simulink model "tqdtqr_rebuild_V3"  (R2021b)
settings: Solver=VariableStepAuto  StartTime=0.0  StopTime=10.0  RelTol=1e-3
undefined symbols (not defined in the file): ATQD_AfterTqMinGain_X_Deg, ATQD_APSCreepBaseTqD_X_kph, ATQD_APSCreepBaseTqD_Y_Deg, ATQD_APSCreepBaseTqR_X_kph, ATQD_APSCreepBaseTqR_Y_Deg, ATQD_APSCreepIterm_X_kph, ATQD_APSCreepIterm_Y_kph, ATQD_APSCreepPterm_X_kph, ATQD_APSCreepPterm_Y_kph, ATQD_APSDecReq_X_kph, ATQD_APSDecReq_Y_mps2, ATQD_APSDecReqCMD_X_kph, ATQD_APSDecReqTs_X_pct, ATQD_APSDecTimeGain_X_Deg, ATQD_APSDecTimeGain_Y_s, ATQD_APSReqLowSpd_X_Deg, ATQD_AutoHoldReleaseBPS_X_Deg, ATQD_AWDLoadTrqnsGain_X_kg, ATQD_AWDLoadTrqnsGain_Y_pct, ATQD_BOSEnBPSPosn_X_kph, ATQD_BOSMap_X_rpm, ATQD_BOSMap_Y_pct, ATQD_CreepBaseTqD_X_kph, ATQD_CreepBaseTqD_Y_Deg, ATQD_CreepBaseTqR_X_kph, ATQD_CreepBaseTqR_Y_Deg, ATQD_CreepBPSDisPosn_X_Deg, ATQD_CreepBPSDisPosnR_X_Deg, ATQD_CreepBPSEnPosn_X_Deg, ATQD_CreepBPSEnPosnR_X_Deg, ATQD_CreepDeltaTq_X_kph, ATQD_CreepIterm_X_kph, ATQD_CreepIterm_Y_kph, ATQD_CreepItermMaxLimit_X_pct, ATQD_CreepPreloadTime_X_kph, ATQD_CreepPreloadTq_X_kph, ATQD_CreepPreloadTq_Y_s, ATQD_CreepProtTq_X_Deg, ATQD_CreepPterm_X_kph, ATQD_CreepPterm_Y_kph, ATQD_CreepRrTqSpRat_X_rpm, ATQD_CreepRrTqSpRat_Y_Nm, ATQD_CreepTargetSpdD_X_pct, ATQD_CreepTargetSpdR_X_pct, ATQD_CreepUpLimitTq_X_rpm, ATQD_DecIneOPDHoldEnDelay_X_Deg, ATQD_DecIneOPDHoldEnDelay_Y_bar, ATQD_ECOTqMapD_X_rpm, ATQD_ECOTqMapD_Y_pct, ATQD_EMTqMapD_X_rpm, ATQD_EMTqMapD_Y_pct, ATQD_EOPDTqMapDCon_X_rpm, ATQD_EOPDTqMapDCon_Y_Deg, ATQD_EstInitVehWeight_X_c, ATQD_FAfterTqCMDGain_X_rpm, ATQD_FAfterTqCMDGain_Y_pct, ATQD_ForceLowSpd_X_Deg, ATQD_ForcePLimitSpd_X_Deg, ATQD_FrLossMAPLowV_X_rpm, ATQD_FrLossMAPLowV_Y_Nm ... (+949)
libraries: simulink x235, hcu_lib x208, tqr x63, tqd x6
(part 25 of 37)

== system tqdtqr_rebuild_V3/Input_Convert/Signal function/combo key/Mode Coordination ==
  VSCP_StreetFightMode_flg : Inport
  VSCP_EngineeringMode_flg : Inport  Port=2
  VSCP_ManufactureMode_flg : Inport  Port=3
  VSCP_ExhibitionMode_flg : Inport  Port=4
  VSCP_DiagnosisOffMode_flg : Inport  Port=5
  DiagnosisOff : Subsystem  TreatAsAtomicUnit=on
  Engineering : Subsystem  TreatAsAtomicUnit=on
  Exhibition : Subsystem  TreatAsAtomicUnit=on
  If : If  NumInputs=5  IfExpression=u1 ~=0  ElseIfExpressions=u2 ~= 0, u3 ~= 0, u4 ~= 0, u5 ~= 0
  Manufacture : Subsystem  TreatAsAtomicUnit=on
  Merge : Merge  Inputs=6
  Product : Subsystem  TreatAsAtomicUnit=on
  StreetFight : Subsystem  TreatAsAtomicUnit=on
  VSCP_SysMode_enum : Outport
  wires:
  [VSCP_ManufactureMode_flg] -> If/3
  [VSCP_StreetFightMode_flg] -> If/1
  [VSCP_DiagnosisOffMode_flg] -> If/5
  [VSCP_ExhibitionMode_flg] -> If/4
  [VSCP_EngineeringMode_flg] -> If/2
  VSCP_StreetFightMode_flg/1 -> [VSCP_StreetFightMode_flg]
  VSCP_EngineeringMode_flg/1 -> [VSCP_EngineeringMode_flg]
  VSCP_ManufactureMode_flg/1 -> [VSCP_ManufactureMode_flg]
  VSCP_ExhibitionMode_flg/1 -> [VSCP_ExhibitionMode_flg]
  VSCP_DiagnosisOffMode_flg/1 -> [VSCP_DiagnosisOffMode_flg]
  If/1 -> StreetFight/Action
  If/2 -> Engineering/Action
  If/6 -> Product/Action
  If/3 -> Manufacture/Action
  If/4 -> Exhibition/Action
  If/5 -> DiagnosisOff/Action
  StreetFight/1(StreetFight) -> Merge/1
  Engineering/1(Engineering) -> Merge/2
  Manufacture/1(Manufacture) -> Merge/3
  Exhibition/1(Exhibition) -> Merge/4
  DiagnosisOff/1(DiagnosisOff) -> Merge/5
  Product/1(Product) -> Merge/6
  Merge/1 -> [VSCP_SysMode_enum]  "VTQD_SysMode_enum"
  [VSCP_SysMode_enum] -> VSCP_SysMode_enum/1

== system tqdtqr_rebuild_V3/Input_Convert/Signal function/combo key/Operation Condition ==
  VINP_PwrSta_enum : Inport
  VINP_ShiftGearPosn_enum : Inport  Port=2
  VSCP_ComboKeyEnCMD_flg : Inport  Port=3
  AND : Logic  AllPortsSameDT=off  OutDataTypeStr=boolean
  AND1 : Logic  AllPortsSameDT=off  OutDataTypeStr=boolean
  Constant1 : Constant  Value=ENUM_POWERSTA_ON
  Constant2 : Constant  Value=ENUM_POWERSTA_READY
  Constant3 : Constant  Value=ENUM_GEARPOSNTOCAN_N
  Constant4 : Constant  Value=ENUM_GEARPOSNTOCAN_P
  Equal{,1..3} (4 alike) : RelationalOperator  Operator===  OutDataTypeStr=boolean  RndMeth=Simplest
  OR : Logic  Operator=OR  AllPortsSameDT=off  OutDataTypeStr=boolean
  OR1 : Logic  Operator=OR  AllPortsSameDT=off  OutDataTypeStr=boolean
  VSCP_ComboKeyPreEn_flg : Outport
  VSCP_ComboKeyEn_flg : Outport  Port=2
  wires:
  OR/1 -> AND/1
  Equal2/1 -> OR1/1
  Constant3/1 -> Equal3/2
  Equal/1 -> OR/1
  [VINP_ShiftGearPosn_enum] -> Equal2/1
  Constant1/1 -> Equal1/2
  Equal3/1 -> OR1/2
  Constant4/1 -> Equal2/2
  [VINP_ShiftGearPosn_enum] -> Equal3/1
  [VINP_PwrSta_enum] -> Equal/1
  Constant2/1 -> Equal/2
  [VINP_PwrSta_enum] -> Equal1/1
  Equal1/1 -> OR/2
  OR1/1 -> AND/2
  VINP_PwrSta_enum/1 -> [VINP_PwrSta_enum]
  VINP_ShiftGearPosn_enum/1 -> [VINP_ShiftGearPosn_enum]
  [VSCP_ComboKeyPreEn_flg] -> VSCP_ComboKeyPreEn_flg/1
  AND/1 -> [VSCP_ComboKeyPreEn_flg]  "VTQD_ComboKeyPreEn_flg"
  VSCP_ComboKeyEnCMD_flg/1 -> [VSCP_ComboKeyEnCMD_flg]
  [VSCP_ComboKeyPreEn_flg] -> AND1/1
  [VSCP_ComboKeyEnCMD_flg] -> AND1/2
  AND1/1 -> [VSCP_ComboKeyEn_flg]  "VTQD_ComboKeyEn_flg"
  [VSCP_ComboKeyEn_flg] -> VSCP_ComboKeyEn_flg/1

== system tqdtqr_rebuild_V3/Input_Convert/Signal function/combo key/Signal Status Detection ==
  note: Button result -> combo key command
  note: Button status
  note: Button result -> combo key value
  note: Button status
  note: Combo Key Note:
      | ENUM_COMBOKEY_NONE = uint8(0); None
      | ENUM_COMBOKEY_REGENDOWN = uint8(1); VINP_SWC2RegenDown_flg
      | ENUM_COMBOKEY_REGENUP = uint8(2); VINP_SWC2RegenUp_flg
      | ENUM_COMBOKEY_RESUP = uint8(3); VINP_SWC2LScrollUpSta_flg
      | ENUM_COMBOKEY_SETDOWN = uint8(4); VINP_SWC2LScrollDownSta_flg
      | ENUM_COMBOKEY_SWCUP = uint8(5); VINP_SWC2RScrollUpSta_flg
      | ENUM_COMBOKEY_SWCDOWN = uint8(6); VINP_SWC2RScrollDownSta_flg
      | ENUM_COMBOKEY_CANCEL = uint8(7); VINP_SWC2LScrollPressSta_flg
      | ENUM_COMBOKEY_SWCACC = uint8(8); VINP_SWC2LADASSta_flg
      | ENUM_COMBOKEY_DISTANCE = uint8(9); VINP_SWC2LDriveModeSta_flg
      | ENUM_COMBOKEY_SWCMODE = uint8(10); VINP_SWC2RScrollPressSta_flg
      | ENUM_COMBOKEY_SWCRIGHT = uint8(11); VINP_SWC2RRightSta_flg
      | ENUM_COMBOKEY_SWCLEFT = uint8(12); VINP_SWC2RLeftSta_flg
  TASK_TIME_10_MS : Inport
  VINP_SWCRegenDown_flg : Inport  Port=2
  VINP_SWCRegenUp_flg : Inport  Port=3
  VINP_SWCResUpSta_flg : Inport  Port=4
  VINP_SWCSetdownSta_flg : Inport  Port=5
  VINP_SWCUpSta_flg : Inport  Port=6
  VINP_SWCDownSta_flg : Inport  Port=7
  VINP_SWCCANCELSta_flg : Inport  Port=8
  VSCP_ComboKeyPreEn_flg : Inport  Port=9
  VINP_SWCACCSta_flg : Inport  Port=10
  VSCP_SysMode_enum : Inport  Port=11
  VINP_SWCDistanceSta_flg : Inport  Port=12
  VINP_SWCmodeSta_flg : Inport  Port=13
  VINP_SWCRightSta_flg : Inport  Port=14
  VINP_SWCLeftSta_flg : Inport  Port=15
  VSCP_ComboKeyEn_flg : Inport  Port=16
  AND{,1..14} (15 alike) : Logic  AllPortsSameDT=off  OutDataTypeStr=boolean
  Constant{,1..5,10..15} (12 alike) : Constant  Value=KTQD_SetSpdShortPLim_s
  Constant{6..9} (4 alike) : Constant  Value=KTQD_ComboKeyLongDet_s
  Delay : Delay  DelayLength=1
  DelayEnable{,1..15} (16 alike) : hcu_lib/Basic_Blocks/DelayEnable
  Detect Decrease{,1..5,10..15} (12 alike) : simulink/Logic and Bit Operations/Detect Decrease  vinit=boolean(0)  OutDataTypeStr=boolean
  Detect Decrease{6..9} (4 alike) : simulink/Logic and Bit Operations/Detect Decrease  vinit=0.0  OutDataTypeStr=boolean
  If : If  NumInputs=12  IfExpression=u1~=0  ElseIfExpressions=u2~=0,u3~=0,u4~=0,u5~=0,u6~=0,u7 ~=0,u8~=0,u9~=0,u10~=0,u11~=0,u12~=0
  Merge : Merge  Inputs=13
  None : Subsystem  TreatAsAtomicUnit=on
  SR_Latch : hcu_lib/Basic_Blocks/SR_Latch
  SWCACCSta : Subsystem  TreatAsAtomicUnit=on
  SWCCANCELStaShort : Subsystem  TreatAsAtomicUnit=on
  SWCDistanceSta : Subsystem  TreatAsAtomicUnit=on
  SWCDownStaShort : Subsystem  TreatAsAtomicUnit=on
  SWCLeftSta : Subsystem  TreatAsAtomicUnit=on
  SWCRegenDownShort : Subsystem  TreatAsAtomicUnit=on
  SWCRegenUpShort : Subsystem  TreatAsAtomicUnit=on
  SWCResUpStaShort : Subsystem  TreatAsAtomicUnit=on
  SWCRightSta : Subsystem  TreatAsAtomicUnit=on
  SWCSetdownStaShort : Subsystem  TreatAsAtomicUnit=on
  SWCUpStaShort : Subsystem  TreatAsAtomicUnit=on
  SWCmodeSta : Subsystem  TreatAsAtomicUnit=on
  Street Fight Switch Off : Subsystem
  VSCP_ComboKey_enum : Outport
  VSCP_ComboKeyEnCMD_flg : Outport  Port=2
  VSCP_ComboKeyReset_flg : Outport  Port=3
  VSCP_ComboKeyEnter_flg : Outport  Port=4
  VSCP_StreetFightModeOff_flg : Outport  Port=5
  wires:
  [VSCP_ComboKey_enum] -> VSCP_ComboKey_enum/1
  Constant/1 -> DelayEnable/2
  SWCRegenUpShort/1(SWCRegenUpShort_enum) -> [SWCRegenUpShort_enum]
  [SWCUpStaShort_enum] -> Merge/5
  VINP_SWCResUpSta_flg/1 -> [VINP_SWCResUpSta_flg]
  [VINP_SWCSetdownSta_flg] -> DelayEnable3/1
  SWCUpStaShort/1(SWCUpStaShort_enum) -> [SWCUpStaShort_enum]
  Detect Decrease3/1 -> [VSCP_SWCSetdownStaShort_flg]  "VTQD_SWCSetdownStaShort_flg"
  Detect Decrease5/1 -> [VSCP_SWCDownStaShort_flg]  "VTQD_SWCDownStaShort_flg"
  If/2 -> SWCRegenUpShort/Action
  Constant2/1 -> DelayEnable2/2
  DelayEnable4/1 -> Detect Decrease4/1
  Detect Decrease4/1 -> [VSCP_SWCUpStaShort_flg]  "VTQD_SWCUpStaShort_flg"
  DelayEnable5/1 -> Detect Decrease5/1
  Constant5/1 -> DelayEnable5/2
  If/6 -> SWCDownStaShort/Action
  [TASK_TIME_10_MS] -> DelayEnable3/3
  [SWCSetdownStaShort_enum] -> Merge/4
  [TASK_TIME_10_MS] -> DelayEnable5/3
  Constant3/1 -> DelayEnable3/2
  VINP_SWCRegenDown_flg/1 -> [VINP_SWCRegenDown_flg]
  [SWCResUpStaShort_enum] -> Merge/3
  DelayEnable3/1 -> Detect Decrease3/1
  [VINP_SWCDownSta_flg] -> DelayEnable5/1
  If/5 -> SWCUpStaShort/Action
  Detect Decrease/1 -> [VSCP_SWCRegenDownShort_flg]  "VTQD_SWCRegenDownShort_flg"
  TASK_TIME_10_MS/1 -> [TASK_TIME_10_MS]
  [TASK_TIME_10_MS] -> DelayEnable4/3
  If/13 -> None/Action
  Detect Decrease2/1 -> [VSCP_SWCResUpStaShort_flg]  "VTQD_SWCResUpStaShort_flg"
  If/4 -> SWCSetdownStaShort/Action
  Detect Decrease1/1 -> [VSCP_SWCRegenUpShort_flg]  "VTQD_SWCRegenUpShort_flg"
  VINP_SWCDownSta_flg/1 -> [VINP_SWCDownSta_flg]
  [VINP_SWCUpSta_flg] -> DelayEnable4/1
  Constant4/1 -> DelayEnable4/2
  [SWCRegenUpShort_enum] -> Merge/2
  If/1 -> SWCRegenDownShort/Action
  Constant1/1 -> DelayEnable1/2
  [TASK_TIME_10_MS] -> DelayEnable/3
  VINP_SWCSetdownSta_flg/1 -> [VINP_SWCSetdownSta_flg]
  [VINP_SWCRegenDown_flg] -> DelayEnable/1
  [SWCDownStaShort_enum] -> Merge/6
  VINP_SWCRegenUp_flg/1 -> [VINP_SWCRegenUp_flg]
  DelayEnable/1 -> Detect Decrease/1
  [VINP_SWCResUpSta_flg] -> DelayEnable2/1
  [TASK_TIME_10_MS] -> DelayEnable2/3
  DelayEnable2/1 -> Detect Decrease2/1
  VINP_SWCUpSta_flg/1 -> [VINP_SWCUpSta_flg]
  [SWCRegenDownShort_enum] -> Merge/1
  None/1(None_enum) -> [None_enum]
  [VINP_SWCRegenUp_flg] -> DelayEnable1/1
  [TASK_TIME_10_MS] -> DelayEnable1/3
  DelayEnable1/1 -> Detect Decrease1/1
  If/3 -> SWCResUpStaShort/Action
  SWCRegenDownShort/1(SWCRegenDownShort_enum) -> [SWCRegenDownShort_enum]
  SWCResUpStaShort/1(SWCResUpStaShort_enum) -> [SWCResUpStaShort_enum]
  SWCSetdownStaShort/1(SWCSetdownStaShort_enum) -> [SWCSetdownStaShort_enum]
  Merge/1 -> [VSCP_ComboKey_enum]  "VTQD_ComboKey_enum"
  SWCDownStaShort/1(SWCDownStaShort_enum) -> [SWCDownStaShort_enum]
  [VINP_SWCRegenDown_flg] -> DelayEnable6/1
  [TASK_TIME_10_MS] -> DelayEnable6/3
  Constant6/1 -> DelayEnable6/2
  DelayEnable6/1 -> [VSCP_SWCRegenDownLong_flg]  "VTQD_SWCRegenDownLong_flg"
  DelayEnable7/1 -> [VSCP_SWCRegenUpLong_flg]  "VTQD_SWCRegenUpLong_flg"
  Constant7/1 -> DelayEnable7/2
  [TASK_TIME_10_MS] -> DelayEnable7/3
  [VINP_SWCRegenUp_flg] -> DelayEnable7/1
  [VSCP_SWCRegenDownLong_flg] -> AND/1
  [VSCP_SWCRegenUpLong_flg] -> AND/2
  SR_Latch/1 -> [VSCP_ComboKeyEnCMD_flg]  "VTQD_ComboKeyEnCMD_flg"
  VINP_SWCCANCELSta_flg/1 -> [VINP_SWCCANCELSta_flg]
  [VINP_SWCCANCELSta_flg] -> DelayEnable8/1
  [TASK_TIME_10_MS] -> DelayEnable8/3
  Constant8/1 -> DelayEnable8/2
  DelayEnable8/1 -> [VSCP_SWCCANCELStaLong_flg]  "VTQD_SWCCANCELStaLong_flg"
  [VSCP_ComboKeyEnCMD_flg] -> VSCP_ComboKeyEnCMD_flg/1
  AND/1 -> Detect Decrease6/1
  Detect Decrease6/1 -> SR_Latch/1
  [VSCP_SWCCANCELStaLong_flg] -> Detect Decrease7/1
  Detect Decrease7/1 -> SR_Latch/2
  VSCP_ComboKeyPreEn_flg/1 -> [VSCP_ComboKeyPreEn_flg]
  AND1/1 -> If/1
  [VSCP_ComboKeyPreEn_flg] -> AND1/2
  AND2/1 -> If/2
  [VSCP_ComboKeyPreEn_flg] -> AND2/2
  AND3/1 -> If/3
  [VSCP_SWCResUpStaShort_flg] -> AND3/1
  [VSCP_ComboKeyPreEn_flg] -> AND3/2
  AND4/1 -> If/4
  [VSCP_ComboKeyPreEn_flg] -> AND4/2
  AND5/1 -> If/5
  [VSCP_ComboKeyPreEn_flg] -> AND5/2
  AND6/1 -> If/6
  [VSCP_ComboKeyPreEn_flg] -> AND6/2
  DelayEnable9/1 -> [VSCP_SWCACCStaLong_flg]  "VTQD_SWCACCStaLong_flg"
  Constant9/1 -> DelayEnable9/2
  [TASK_TIME_10_MS] -> DelayEnable9/3
  [VINP_SWCACCSta_flg] -> DelayEnable9/1
  VINP_SWCACCSta_flg/1 -> [VINP_SWCACCSta_flg]
  [VSCP_SWCACCStaLong_flg] -> Detect Decrease8/1
  [VSCP_ComboKeyReset_flg] -> VSCP_ComboKeyReset_flg/1
  [VSCP_SWCCANCELStaLong_flg] -> Detect Decrease9/1
  [VSCP_ComboKeyEnter_flg] -> VSCP_ComboKeyEnter_flg/1
  Detect Decrease8/1 -> AND7/1
  [VSCP_ComboKeyEn_flg] -> AND7/2
  AND7/1 -> [VSCP_ComboKeyReset_flg]  "VTQD_ComboKeyReset_flg"
  Detect Decrease9/1 -> AND8/1
  AND8/1 -> [VSCP_ComboKeyEnter_flg]  "VTQD_ComboKeyEnter_flg"
  [VINP_SWCCANCELSta_flg] -> DelayEnable10/1
  [TASK_TIME_10_MS] -> DelayEnable10/3
  Constant10/1 -> DelayEnable10/2
  DelayEnable10/1 -> Detect Decrease10/1
  Detect Decrease10/1 -> [VSCP_SWCCANCELStaShort_flg]  "VTQD_SWCCANCELStaShort_flg"
  Street Fight Switch Off/1(VSCP_StreetFightModeOff_flg) -> [VSCP_StreetFightModeOff_flg]
  [TASK_TIME_10_MS] -> Street Fight Switch Off/1(TASK_TIME_10_MS)
  [VSCP_SWCCANCELStaShort_flg] -> Street Fight Switch Off/2(VSCP_SWCCANCELStaShort_flg)
  [VSCP_ComboKeyPreEn_flg] -> Street Fight Switch Off/3(VSCP_ComboKeyPreEn_flg)
  [VSCP_SWCCANCELStaLong_flg] -> Street Fight Switch Off/4(SWCCANCELStaLong_flg)
  [VSCP_StreetFightModeOff_flg] -> VSCP_StreetFightModeOff_flg/1
  VSCP_SysMode_enum/1 -> [VSCP_SysMode_enum]
  [VSCP_SysMode_enum] -> Street Fight Switch Off/5(VSCP_SysMode_enum)
  Detect Decrease11/1 -> [VSCP_SWCACCSta_flg]  "VSCP_SWCACCSta_flg"
  DelayEnable11/1 -> Detect Decrease11/1
  Constant11/1 -> DelayEnable11/2
  [TASK_TIME_10_MS] -> DelayEnable11/3
  [VINP_SWCACCSta_flg] -> DelayEnable11/1
  [VSCP_ComboKeyPreEn_flg] -> AND9/2
  AND9/1 -> If/7
  SWCCANCELStaShort/1(SWCCANCELStaShort_enum) -> [SWCCANCELStaShort_enum]
  If/7 -> SWCCANCELStaShort/Action
  [VSCP_ComboKeyPreEn_flg] -> AND10/2
  AND10/1 -> If/8
  SWCACCSta/1(SWCACCSta_enum) -> [SWCACCSta_enum]
  If/8 -> SWCACCSta/Action
  VINP_SWCDistanceSta_flg/1 -> [VINP_SWCDistanceSta_flg]
  [VINP_SWCDistanceSta_flg] -> DelayEnable12/1
  [TASK_TIME_10_MS] -> DelayEnable12/3
  Constant12/1 -> DelayEnable12/2
  DelayEnable12/1 -> Detect Decrease12/1
  Detect Decrease12/1 -> [VSCP_SWCDistanceSta_flg]  "VTQD_SWCDistanceSta_flg"
  [VSCP_ComboKeyPreEn_flg] -> AND11/2
  AND11/1 -> If/9
  If/9 -> SWCDistanceSta/Action
  SWCDistanceSta/1(SWCDownStaShort_enum) -> [SWCDistanceSta_enum]
  VINP_SWCmodeSta_flg/1 -> [VINP_SWCmodeSta_flg]
  Detect Decrease13/1 -> [VSCP_SWCmodeSta_flg]  "VTQD_SWCmodeSta_flg"
  DelayEnable13/1 -> Detect Decrease13/1
  Constant13/1 -> DelayEnable13/2
  [TASK_TIME_10_MS] -> DelayEnable13/3
  [VINP_SWCmodeSta_flg] -> DelayEnable13/1
  [VSCP_ComboKeyPreEn_flg] -> AND12/2
  AND12/1 -> If/10
  If/10 -> SWCmodeSta/Action
  SWCmodeSta/1(SWCmodeSta_enum) -> [SWCmodeSta_enum]
  VINP_SWCRightSta_flg/1 -> [VINP_SWCRightSta_flg]
  [VINP_SWCRightSta_flg] -> DelayEnable14/1
  [TASK_TIME_10_MS] -> DelayEnable14/3
  Constant14/1 -> DelayEnable14/2
  DelayEnable14/1 -> Detect Decrease14/1
  Detect Decrease14/1 -> [VSCP_SWCRightSta_flg]  "VTQD_SWCRightSta_flg"
  [VSCP_ComboKeyPreEn_flg] -> AND13/2
  AND13/1 -> If/11
  If/11 -> SWCRightSta/Action
  SWCRightSta/1(SWCRightSta_enum) -> [SWCRightSta_enum]
  VINP_SWCLeftSta_flg/1 -> [VINP_SWCLeftSta_flg]
  Detect Decrease15/1 -> [VSCP_SWCLeftSta_flg]  "VTQD_SWCLeftSta_flg"
  DelayEnable15/1 -> Detect Decrease15/1
  Constant15/1 -> DelayEnable15/2
  [TASK_TIME_10_MS] -> DelayEnable15/3
  [VINP_SWCLeftSta_flg] -> DelayEnable15/1
  [VSCP_ComboKeyPreEn_flg] -> AND14/2
  AND14/1 -> If/12
  If/12 -> SWCLeftSta/Action
  SWCLeftSta/1(SWCLeftSta_enum) -> [SWCLeftSta_enum]
  [None_enum] -> Merge/13
  [SWCCANCELStaShort_enum] -> Merge/7
  [SWCACCSta_enum] -> Merge/8
  [SWCDistanceSta_enum] -> Merge/9
  [SWCmodeSta_enum] -> Merge/10
  [SWCRightSta_enum] -> Merge/11
  [SWCLeftSta_enum] -> Merge/12
  [VSCP_SWCRegenDownShort_flg] -> AND1/1
  [VSCP_SWCRegenUpShort_flg] -> AND2/1
  [VSCP_SWCSetdownStaShort_flg] -> AND4/1
  [VSCP_SWCUpStaShort_flg] -> AND5/1
  [VSCP_SWCDownStaShort_flg] -> AND6/1
  [VSCP_SWCCANCELStaShort_flg] -> AND9/1
  [VSCP_SWCACCSta_flg] -> AND10/1
  [VSCP_SWCDistanceSta_flg] -> AND11/1
  [VSCP_SWCmodeSta_flg] -> AND12/1
  [VSCP_SWCRightSta_flg] -> AND13/1
  [VSCP_SWCLeftSta_flg] -> AND14/1
  VSCP_ComboKeyEn_flg/1 -> [VSCP_ComboKeyEn_flg]
  Delay/1 -> AND8/2
  [VSCP_ComboKeyEn_flg] -> Delay/1

== system tqdtqr_rebuild_V3/Input_Convert/Main function/AvaliableTqLimit function/TorqueCapacityCalcalation/CapacityDistribution ==
  VTQD_FrEDUSpRat_cmd : Inport
  VTQD_RrEDUSpRat_rat : Inport  Port=2
  VTQD_TMPwrAvailDchrg_kW : Inport  Port=3
  VINP_HVBPwrAvailChrg_kw : Inport  Port=4
  VTQD_MotorLossTotal_kw : Inport  Port=5
  Abs1 : Abs
  Add : Sum  Inputs=+-
  Constant12 : Constant  Value=ZERO_FLOAT
  Max : MinMax  Function=max  Inputs=2
  Product{,1,4..5} (4 alike) : Product
  VTQD_FrHVBPwrAvailDchrg_kw : Outport
  VTQD_RrHVBPwrAvailDchrg_kw : Outport  Port=2
  VTQD_FrHVBPwrAvailChrg_kw : Outport  Port=3
  VTQD_RrHVBPwrAvailChrg_kw : Outport  Port=4
  wires:
  VTQD_RrEDUSpRat_rat/1 -> [VTQD_RrEDUSpRat_rat]
  VTQD_FrEDUSpRat_cmd/1 -> [VTQD_FrEDUSpRat_rat]
  VINP_HVBPwrAvailChrg_kw/1 -> Abs1/1
  Product4/1 -> VTQD_FrHVBPwrAvailChrg_kw/1
  Product5/1 -> VTQD_RrHVBPwrAvailChrg_kw/1
  Product1/1 -> VTQD_RrHVBPwrAvailDchrg_kw/1  "VTQD_RrHVBPwrAvailDchrg_kW"
  [VTQD_FrEDUSpRat_rat] -> Product4/1
  [VTQD_FrEDUSpRat_rat] -> Product/1
  Abs1/1 -> Product4/2, Product5/1
  [VTQD_RrEDUSpRat_rat] -> Product5/2
  Product/1 -> VTQD_FrHVBPwrAvailDchrg_kw/1  "VTQD_FrHVBPwrAvailDchrg_kW"
  [VTQD_RrEDUSpRat_rat] -> Product1/2
  VTQD_TMPwrAvailDchrg_kW/1 -> Add/1
  VTQD_MotorLossTotal_kw/1 -> Add/2
  Add/1 -> Max/1
  Constant12/1 -> Max/2
  Max/1 -> Product1/1, Product/2

== system tqdtqr_rebuild_V3/Input_Convert/Main function/AvaliableTqLimit function/TorqueCapacityCalcalation/MOTOR Loss MAP  ==
  note: Rear Loss Power Calculation
  note: Calabration Parameters/Maps
  note: Front Loss Power Calculation
  note: Determination
  VTQD_FrShaftSpd_rpm : Inport
  VTQD_RrShaftSpd_rpm : Inport  Port=2
  VTQD_CoordWhlTqDemFr_Nm : Inport  Port=3
  VTQD_CoordWhlTqDemRr_Nm : Inport  Port=4
  VINP_FrMCUDCBusVolt_V : Inport  Port=5
  VINP_RrMCUDCBusVolt_V : Inport  Port=6
  VPMM_DrivetrainSelect_enum : Inport  Port=7
  AND : Logic  AllPortsSameDT=off  OutDataTypeStr=boolean
  AND2 : Logic  AllPortsSameDT=off  OutDataTypeStr=boolean
  Add : Sum
  Add2 : Sum
  Add3 : Sum
  Constant : Constant  Value=KTQD_FrLossMAPLowV_V
  Constant1 : Constant  Value=KTQD_FrLossMAPHighV_V
  Constant10 : Constant  Value=eps  OutDataTypeStr=single
  Constant{6,11..13} (4 alike) : Constant  Value=ZERO_FLOAT
  Constant2 : Constant  Value=KTQD_RrLossMAPLowV_V
  Constant3 : Constant  Value=KTQD_RrLossMAPHighV_V
  Constant4 : Constant  Value=ENUM_DRIVETRAIN_AWD
  Constant5 : Constant  Value=ENUM_DRIVETRAIN_RWD
  Constant7 : Constant  Value=eps  OutDataTypeStr=single
  Divide : Product  Inputs=*/
  Divide2 : Product  Inputs=*/
  Equal : RelationalOperator  Operator===  OutDataTypeStr=boolean  RndMeth=Simplest
  Equal1 : RelationalOperator  Operator===  OutDataTypeStr=boolean  RndMeth=Simplest
  GreaterThan : RelationalOperator  Operator=>  OutDataTypeStr=boolean  RndMeth=Simplest
  GreaterThan2 : RelationalOperator  Operator=>  OutDataTypeStr=boolean  RndMeth=Simplest
  Less Than : RelationalOperator  Operator=<  OutDataTypeStr=boolean  RndMeth=Simplest
  Less Than2 : RelationalOperator  Operator=<  OutDataTypeStr=boolean  RndMeth=Simplest
  MTQD_FrLossMAPHighV_Z_kW : Lookup_n-D  BreakpointsForDimension1=ATQD_FrLossMAPLowV_Y_Nm  BreakpointsForDimension2=ATQD_FrLossMAPLowV_X_rpm  Table=MTQD_FrLossMAPHighV_Z_kW  InternalRulePriority=Speed  RndMeth=Simplest  InputSameDT=on
      settings: InputPortMap=u0,u1
  MTQD_FrLossMAPLowV_Z_kW : Lookup_n-D  BreakpointsForDimension1=ATQD_FrLossMAPLowV_Y_Nm  BreakpointsForDimension2=ATQD_FrLossMAPLowV_X_rpm  Table=MTQD_FrLossMAPLowV_Z_kW  InternalRulePriority=Speed  RndMeth=Simplest  InputSameDT=on
      settings: InputPortMap=u0,u1
  MTQD_RrLossMAPHighV_Z_kW : Lookup_n-D  BreakpointsForDimension1=ATQD_RrLossMAPLowV_Y_Nm  BreakpointsForDimension2=ATQD_RrLossMAPLowV_X_rpm  Table=MTQD_RrLossMAPHighV_Z_kW  InternalRulePriority=Speed  RndMeth=Simplest  InputSameDT=on
      settings: InputPortMap=u0,u1
  MTQD_RrLossMAPLowV_Z_kW : Lookup_n-D  BreakpointsForDimension1=ATQD_RrLossMAPLowV_Y_Nm  BreakpointsForDimension2=ATQD_RrLossMAPLowV_X_rpm  Table=MTQD_RrLossMAPLowV_Z_kW  InternalRulePriority=Speed  RndMeth=Simplest  InputSameDT=on
      settings: InputPortMap=u0,u1
  Max : MinMax  Function=max  Inputs=2
  Max1 : MinMax  Function=max  Inputs=2
  Product : Product
  Product2 : Product
  Subtract{,1..2,6..8} (6 alike) : Sum  Inputs=+-
  Switch : Switch  Criteria=u2 > Threshold
  Switch1 : Switch  Criteria=u2 > Threshold
  Switch3 : Switch  Criteria=u2 ~= 0
  Switch4 : Switch  Criteria=u2 ~= 0
  VTQD_MotorLossTotal_kW : Outport
  wires:
  VINP_FrMCUDCBusVolt_V/1 -> [VINP_FrMCUDCBusVolt_V]
  VINP_RrMCUDCBusVolt_V/1 -> [VINP_RrMCUDCBusVolt_V]
  VTQD_CoordWhlTqDemFr_Nm/1 -> [VTQD_CoordWhlTqDemFr_Nm]
  VTQD_FrShaftSpd_rpm/1 -> [VTQD_FrShaftSpd_rpm]
  VTQD_RrShaftSpd_rpm/1 -> [VTQD_RrShaftSpd_rpm]
  VTQD_CoordWhlTqDemRr_Nm/1 -> [VTQD_CoordWhlTqDemRr_Nm]
  VPMM_DrivetrainSelect_enum/1 -> [VPMM_DrivetrainSelect_enum]
  MTQD_FrLossMAPLowV_Z_kW/1 -> [VTQD_FrLossMAPLowV_kW]  "VTQD_FrLossMAPLowV_kW"
  [VTQD_RrShaftSpd_rpm] -> MTQD_RrLossMAPHighV_Z_kW/2
  Switch/1 -> [VTQD_MotorLossTotal_kW]  "VTQD_MotorLossTotal_kW"
  Add/1 -> Switch3/1
  Constant2/1 -> [VTQD_RrLossMAPLowV_V]  "VTQD_RrLossMAPLowV_V"
  Constant7/1 -> Max1/2
  Subtract/1 -> Divide/1
  Constant1/1 -> [VTQD_FrLossMAPHighV_V]  "VTQD_FrLossMAPHighV_V"
  [VTQD_RrShaftSpd_rpm] -> MTQD_RrLossMAPLowV_Z_kW/2
  Subtract8/1 -> Product2/2
  Constant3/1 -> [VTQD_RrLossMAPHighV_V]  "VTQD_RrLossMAPHighV_V"
  Subtract1/1 -> Max/1
  Constant/1 -> [VTQD_FrLossMAPLowV_V]  "VTQD_FrLossMAPLowV_V"
  [VTQD_FrLossMAPLowV_V] -> Subtract/2
  [VTQD_RrLossMAPLowV_kW] -> Subtract8/2
  Add2/1 -> Switch/1
  [VINP_RrMCUDCBusVolt_V] -> Less Than2/1
  MTQD_RrLossMAPHighV_Z_kW/1 -> [VTQD_RrLossMAPHighV_kW]  "VTQD_RrLossMAPHighV_kW"
  Switch3/1 -> [VTQD_FrLossMAPFinal_kW]  "VTQD_FrLossMAPFinal_kW"
  [VTQD_CoordWhlTqDemRr_Nm] -> GreaterThan2/1
  [VTQD_RrLossMAPHighV_kW] -> Subtract8/1
  Product/1 -> Add/1
  Divide/1 -> Product/1
  [VPMM_DrivetrainSelect_enum] -> Equal/1
  [VINP_FrMCUDCBusVolt_V] -> Subtract/1
  Max1/1 -> Divide2/2
  [VTQD_FrLossMAPLowV_kW] -> Add/2
  [VTQD_RrLossMAPHighV_V] -> Less Than2/2
  Constant4/1 -> Equal/2
  Less Than/1 -> AND/2
  [VTQD_RrLossMAPLowV_kW] -> Add3/2
  [VPMM_DrivetrainSelect_enum] -> Equal1/1
  [VINP_FrMCUDCBusVolt_V] -> Less Than/1
  Equal1/1 -> Switch1/2
  [VTQD_CoordWhlTqDemFr_Nm] -> GreaterThan/1
  GreaterThan/1 -> AND/1
  Equal/1 -> Switch/2
  AND2/1 -> Switch4/2
  Subtract2/1 -> Product/2
  [VTQD_CoordWhlTqDemFr_Nm] -> MTQD_FrLossMAPLowV_Z_kW/1
  Constant11/1 -> Switch3/3
  [VTQD_FrLossMAPHighV_kW] -> Subtract2/1
  AND/1 -> Switch3/2
  [VTQD_FrLossMAPHighV_V] -> Subtract1/1
  [VTQD_CoordWhlTqDemFr_Nm] -> MTQD_FrLossMAPHighV_Z_kW/1
  Constant10/1 -> Max/2
  [VTQD_CoordWhlTqDemRr_Nm] -> MTQD_RrLossMAPLowV_Z_kW/1
  [VTQD_CoordWhlTqDemRr_Nm] -> MTQD_RrLossMAPHighV_Z_kW/1
  MTQD_RrLossMAPLowV_Z_kW/1 -> [VTQD_RrLossMAPLowV_kW]  "VTQD_RrLossMAPLowV_kW"
  [VTQD_FrShaftSpd_rpm] -> MTQD_FrLossMAPHighV_Z_kW/2
  Constant13/1 -> GreaterThan2/2
  [VTQD_FrShaftSpd_rpm] -> MTQD_FrLossMAPLowV_Z_kW/2
  [VTQD_RrLossMAPHighV_V] -> Subtract7/1
  Constant6/1 -> GreaterThan/2
  [VTQD_FrLossMAPLowV_V] -> Subtract1/2
  Max/1 -> Divide/2
  [VTQD_FrLossMAPLowV_kW] -> Subtract2/2
  [VTQD_FrLossMAPFinal_kW] -> Switch1/3
  Subtract7/1 -> Max1/1
  [VTQD_FrLossMAPHighV_V] -> Less Than/2
  [VTQD_RrLossMAPLowV_V] -> Subtract7/2
  Add3/1 -> Switch4/1
  Product2/1 -> Add3/1
  Switch1/1 -> Switch/3
  Constant12/1 -> Switch4/3
  Divide2/1 -> Product2/1
  Constant5/1 -> Equal1/2
  [VTQD_RrLossMAPLowV_V] -> Subtract6/2
  Subtract6/1 -> Divide2/1
  [VINP_RrMCUDCBusVolt_V] -> Subtract6/1
  Switch4/1 -> [VTQD_RrLossMAPFinal_kW]  "VTQD_RrLossMAPFinal_kW"
  MTQD_FrLossMAPHighV_Z_kW/1 -> [VTQD_FrLossMAPHighV_kW]  "VTQD_FrLossMAPHighV_kW"
  [VTQD_FrLossMAPFinal_kW] -> Add2/1
  [VTQD_RrLossMAPFinal_kW] -> Switch1/1
  GreaterThan2/1 -> AND2/1
  Less Than2/1 -> AND2/2
  [VTQD_RrLossMAPFinal_kW] -> Add2/2
  [VTQD_MotorLossTotal_kW] -> VTQD_MotorLossTotal_kW/1

== system tqdtqr_rebuild_V3/Input_Convert/Main function/AvaliableTqLimit function/TorqueCapacityCalcalation/TMAvailablePwr_Calculation ==
  VINP_HVBPwrAvailDchrg_kw : Inport
  Add : Sum
  Constant : Constant  Value=KTQD_DCDCCalPwrAvailRsv_kW
  Constant1 : Constant  Value=KTQD_THCMCalPwrAvailRsv_kW
  Constant2 : Constant  Value=KTQD_TMPwrAvailDchrg_kW_ovrdflg
  Constant3 : Constant  Value=ZERO_FLOAT
  Min : MinMax  Function=max  Inputs=2
  Subtract : Sum  Inputs=+-
  Switch : Switch  Criteria=u2 ~= 0
      settings: AttributesFormatString=<%<Criteria>>
  VTQD_TMPwrAvailDchrg_kW : Outport
  wires:
  Constant3/1 -> Min/2
  Min/1 -> Switch/1
  Switch/1 -> VTQD_TMPwrAvailDchrg_kW/1  "VTQD_TMPwrAvailDchrg_kW"
  Constant2/1 -> Switch/2
  Subtract/1 -> Min/1
  Add/1 -> Subtract/2
  VINP_HVBPwrAvailDchrg_kw/1 -> Subtract/1, Switch/3
  Constant1/1 -> Add/2
  Constant/1 -> Add/1

== system tqdtqr_rebuild_V3/Input_Convert/Main function/DriverWhlTqDem function/Creep/If Action Subsystem ==
  In1 : Inport
  Action Port : ActionPort  ActionPortLabel=if(u1 ~= 0)
  Out1 : Outport
  wires:
  In1/1 -> Out1/1

== system tqdtqr_rebuild_V3/Input_Convert/Main function/DriverWhlTqDem function/Creep/If Action Subsystem1 ==
  VTQD_CreepPICtrlReset_flg : Inport
  VTQD_CreepPtermInp_c : Inport  Port=2
  VTQD_CreepItermInp_c : Inport  Port=3
  VTQD_CreepDeltaTq_Nm : Inport  Port=4
  VTQD_ActBPSPosn_pct : Inport  Port=5
  VVMC_APSActive_flg : Inport  Port=6
  Add : Sum
  Add1 : Sum  Inputs=+++
  Constant : Constant  Value=ZERO_FLOAT
  Constant1 : Constant  Value=KTQD_CreepItermMinLimit_Nm
  Constant2 : Constant  Value=KTQD_APSCreepItermMaxLim_Nm
  Constant3 : Constant  Value=ONE_FLOAT
  Constant4 : Constant  Value=ZERO_FLOAT
  Constant5 : Constant  Value=ONE_FLOAT
  Constant87 : Constant  Value=KTQD_APSCreepParOvrd_flg
  Data Type Conversion : DataTypeConversion
  MTQD_CreepItermMaxLimit_Y_Nm : Lookup_n-D  NumberOfTableDimensions=1  BreakpointsForDimension1=ATQD_CreepItermMaxLimit_X_pct  Table=MTQD_CreepItermMaxLimit_Y_Nm  ExtrapMethod=Clip  InternalRulePriority=Speed  RndMeth=Simplest  InputSameDT=on
  OR19 : Logic  Operator=OR  AllPortsSameDT=off  OutDataTypeStr=boolean
  Product : Product
  Product2 : Product
  Saturation Dynamic : simulink/Discontinuities/Saturation Dynamic  OutMin=[]  OutMax=[]  OutDataTypeStr=Inherit: Same as second input  OutDataType=fixdt(1, 16)  OutScaling=2^-10  DoSatur=off
  Switch : Switch  Criteria=u2 ~= 0
      settings: AttributesFormatString=%<Criteria>
  Switch1 : Switch  Criteria=u2 ~= 0
  Switch4 : Switch  Criteria=u2 ~= 0
      settings: AttributesFormatString=%<Criteria>
  Unit Delay : UnitDelay  InitialCondition=boolean(0)  SampleTime=-1  HasFrameUpgradeWarning=on
      settings: AttributesFormatString=%<InitialCondition>
  VTQD_CreepTotalOfstTq_Nm : Outport
  wires:
  Add1/1 -> VTQD_CreepTotalOfstTq_Nm/1  "VTQD_CreepTotalOfstTq_Nm"
  VTQD_CreepDeltaTq_Nm/1 -> [VTQD_CreepDeltaTq_Nm]
  VTQD_CreepItermInp_c/1 -> [VTQD_CreepItermInp_c]
  VTQD_CreepPtermInp_c/1 -> [VTQD_CreepPtermInp_c]
  VTQD_ActBPSPosn_pct/1 -> [VTQD_ActBPSPosn_pct]
  Data Type Conversion/1 -> Add1/3  "VTQD_CreepOffsetTq_Nm"
  Constant1/1 -> Saturation Dynamic/3
  [VTQD_ActBPSPosn_pct] -> MTQD_CreepItermMaxLimit_Y_Nm/1
  [VTQD_CreepPICtrlReset_flg] -> Switch4/2
  Constant/1 -> Switch1/1
  Product/1 -> Switch1/3
  [VTQD_CreepPtermInp_c] -> Product/1
  Constant5/1 -> Product/2
  [VTQD_CreepPICtrlReset_flg] -> Switch1/2
  Add/1 -> Switch4/3
  Switch1/1 -> Add1/1  "VTQD_CreepPtermTq_Nm"
  Saturation Dynamic/1 -> Add1/2  "VTQD_CreepItermTq_Nm"
  Product2/1 -> Add/1
  Switch4/1 -> Unit Delay/1, Saturation Dynamic/2
  Unit Delay/1 -> Add/2
  Constant4/1 -> Switch4/1
  [VTQD_CreepItermInp_c] -> Product2/2
  [VTQD_CreepDeltaTq_Nm] -> Data Type Conversion/1
  VVMC_APSActive_flg/1 -> [VVMC_APSActive_flg]
  MTQD_CreepItermMaxLimit_Y_Nm/1 -> Switch/3
  Switch/1 -> Saturation Dynamic/1  "VTQD_CreepItermMaxLimit_Nm"
  Constant87/1 -> OR19/2
  [VVMC_APSActive_flg] -> OR19/1
  OR19/1 -> Switch/2
  Constant2/1 -> Switch/1
  Constant3/1 -> Product2/1
  VTQD_CreepPICtrlReset_flg/1 -> [VTQD_CreepPICtrlReset_flg]

== system tqdtqr_rebuild_V3/Input_Convert/Main function/DriverWhlTqDem function/Creep/Switch Case Action Subsystem ==
  In1 : Inport
  Action Port : ActionPort  ActionPortLabel=elseif(u2 ~= 0)
  Out1 : Outport
  wires:
  In1/1 -> Out1/1

== system tqdtqr_rebuild_V3/Input_Convert/Main function/DriverWhlTqDem function/Driver mode determination/LHM ==
  VTQD_ActAPSPosn_pct : Inport
  VTQD_TqTargetShaftSpd_rpm : Inport  Port=2
  VTQD_GearActualPosn_enum : Inport  Port=3
  VDDM_VehMalfunLevel_enum : Inport  Port=4
  VVMC_EstSlope_Deg : Inport  Port=5
  VTQD_VehActSpd_kph : Inport  Port=6
  Enable : EnablePort
  Constant : Constant  Value=ZERO_FLOAT
  Constant1 : Constant  Value=ENUM_GEARACTUALPOSN_D
  Constant2 : Constant  Value=ENUM_GEARACTUALPOSN_R
  Constant3 : Constant  Value=ENUM_VEHMALFUNLEVEL_LEVEL2
  Constant5 : Constant  Value=ZERO_FLOAT
  Constant6 : Constant  Value=ZERO_FLOAT
  Equal1 : RelationalOperator  Operator===  OutDataTypeStr=boolean  RndMeth=Simplest
  Equal2 : RelationalOperator  Operator===  OutDataTypeStr=boolean  RndMeth=Simplest
  MTQD_LHMGrade2TqUpLim_Z_Nm : Lookup_n-D  BreakpointsForDimension1=ATQD_LHMGrade2TqUpLim_Y_Deg  BreakpointsForDimension2=ATQD_LHMGrade2TqUpLim_X_kph  Table=MTQD_LHMGrade2TqUpLim_Z_Nm  ExtrapMethod=Clip  InternalRulePriority=Speed  RndMeth=Simplest  InputSameDT=on
      settings: InputPortMap=u0,u1
  MTQD_NL1TqMapD_Z_Nm : Lookup_n-D  BreakpointsForDimension1=ATQD_NL1TqMapD_Y_pct  BreakpointsForDimension2=ATQD_NL1TqMapD_X_rpm  Table=MTQD_NL1TqMapD_Z_Nm  ExtrapMethod=Clip  InternalRulePriority=Speed  RndMeth=Simplest  InputSameDT=on
      settings: InputPortMap=u0,u1
  MTQD_NRMTqMapR_Z_Nm : Lookup_n-D  BreakpointsForDimension1=ATQD_NL1TqMapD_Y_pct  BreakpointsForDimension2=ATQD_NL1TqMapD_X_rpm  Table=MTQD_NRMTqMapR_Z_Nm  ExtrapMethod=Clip  InternalRulePriority=Speed  RndMeth=Simplest  InputSameDT=on
      settings: InputPortMap=u0,u1
  Relational Operator : RelationalOperator  Operator=>  OutDataTypeStr=boolean  RndMeth=Simplest
  Saturation Dynamic : simulink/Discontinuities/Saturation Dynamic  OutMin=[]  OutMax=[]  OutDataTypeStr=Inherit: Same as second input  OutDataType=fixdt(1, 16)  OutScaling=2^-10  DoSatur=off
  Switch1 : Switch  Criteria=u2 ~= 0
      settings: AttributesFormatString=%<Criteria>
  Switch2 : Switch  Criteria=u2 ~= 0
      settings: AttributesFormatString=%<Criteria>
  Switch4 : Switch  Criteria=u2 ~= 0
      settings: AttributesFormatString=%<Criteria>
  VTQD_PedalMapWhlTqLHM_Nm : Outport
  wires:
  VTQD_ActAPSPosn_pct/1 -> [VTQD_ActAPSPosn_pct]
  VTQD_TqTargetShaftSpd_rpm/1 -> [VTQD_TqTargetShaftSpd_rpm]
  VTQD_GearActualPosn_enum/1 -> [VTQD_GearActualPosn_enum]
  VDDM_VehMalfunLevel_enum/1 -> [VDDM_VehMalfunLevel_enum]
  VVMC_EstSlope_Deg/1 -> [VVMC_EstSlope_Deg]
  VTQD_VehActSpd_kph/1 -> [VTQD_VehActSpd_kph]
  [VTQD_TqTargetShaftSpd_rpm] -> MTQD_NL1TqMapD_Z_Nm/2
  [VTQD_GearActualPosn_enum] -> Equal1/1
  [VTQD_LHMPedTqForce0_flg] -> Switch4/2
  MTQD_NRMTqMapR_Z_Nm/1 -> [VTQD_LHMTqMapR_Nm]  "VTQD_LHMTqMapR_Nm"
  [VTQD_VehActSpd_kph] -> MTQD_LHMGrade2TqUpLim_Z_Nm/2
  Relational Operator/1 -> [VTQD_LHMPedTqForce0_flg]  "VTQD_LHMPedTqForce0_flg"
  MTQD_NL1TqMapD_Z_Nm/1 -> [VTQD_LHMTqMapD_Nm]  "VTQD_LHMTqMapD_Nm"
  [VTQD_ActAPSPosn_pct] -> MTQD_NL1TqMapD_Z_Nm/1
  MTQD_LHMGrade2TqUpLim_Z_Nm/1 -> [VTQD_LHMGrade2TqUpLim_Nm]  "VTQD_LHMGrade2TqUpLim_Nm"
  Constant3/1 -> Relational Operator/2
  [VDDM_VehMalfunLevel_enum] -> Relational Operator/1
  [VTQD_LHMTqMapR_Nm] -> Switch2/1
  [VTQD_TqTargetShaftSpd_rpm] -> MTQD_NRMTqMapR_Z_Nm/2
  Switch2/1 -> Switch1/3
  Equal2/1 -> Switch2/2
  [VTQD_GearActualPosn_enum] -> Equal2/1
  Equal1/1 -> Switch1/2
  [VTQD_LHMTqMapD_Nm] -> Switch1/1
  Constant/1 -> Switch2/3
  Constant5/1 -> Saturation Dynamic/3
  [VTQD_ActAPSPosn_pct] -> MTQD_NRMTqMapR_Z_Nm/1
  Constant1/1 -> Equal1/2
  Constant6/1 -> Switch4/1
  Saturation Dynamic/1 -> Switch4/3
  Constant2/1 -> Equal2/2
  Switch4/1 -> VTQD_PedalMapWhlTqLHM_Nm/1
  [VTQD_LHMGrade2TqUpLim_Nm] -> Saturation Dynamic/1
  [VVMC_EstSlope_Deg] -> MTQD_LHMGrade2TqUpLim_Z_Nm/1
  Switch1/1 -> Saturation Dynamic/2

== system tqdtqr_rebuild_V3/Input_Convert/Main function/DriverWhlTqDem function/Driver mode determination/NOLHM ShiftD ECO Invalid ==
  VTQD_RollRegenEnable_flg : Inport
  VTQD_RollingShaftSpd_rpm : Inport  Port=2
  VTQD_TqTargetShaftSpd_rpm : Inport  Port=3
  VTQD_ActAPSPosn_pct : Inport  Port=4
  Enable : EnablePort
  MTQD_ECOTqMapD_Z_Nm : Lookup_n-D  BreakpointsForDimension1=ATQD_ECOTqMapD_Y_pct  BreakpointsForDimension2=ATQD_ECOTqMapD_X_rpm  Table=MTQD_ECOTqMapD_Z_Nm  ExtrapMethod=Clip  InternalRulePriority=Speed  RndMeth=Simplest  InputSameDT=on
      settings: InputPortMap=u0,u1
  MTQD_RollGenMapEL1_Z_Nm : Lookup_n-D  BreakpointsForDimension1=ATQD_RollGenMapEL1_Y_rpm  BreakpointsForDimension2=ATQD_RollGenMapEL1_X_rpm  Table=MTQD_RollGenMapEL1_Z_Nm  ExtrapMethod=Clip  InternalRulePriority=Speed  RndMeth=Simplest  InputSameDT=on
      settings: InputPortMap=u0,u1
  Switch : Switch  Criteria=u2 ~= 0
      settings: AttributesFormatString=%<Criteria>
  VTQD_ELTqMapDOutInv_Nm : Outport
  wires:
  [VTQD_TqTargetShaftSpd_rpm] -> MTQD_RollGenMapEL1_Z_Nm/2
  MTQD_RollGenMapEL1_Z_Nm/1 -> [VTQD_RollGenMapEL1_Nm]
  [VTQD_RollingShaftSpd_rpm] -> MTQD_RollGenMapEL1_Z_Nm/1
  [VTQD_ActAPSPosn_pct] -> MTQD_ECOTqMapD_Z_Nm/1
  [VTQD_TqTargetShaftSpd_rpm] -> MTQD_ECOTqMapD_Z_Nm/2
  MTQD_ECOTqMapD_Z_Nm/1 -> [VTQD_ECOTqMapD_Nm]
  VTQD_TqTargetShaftSpd_rpm/1 -> [VTQD_TqTargetShaftSpd_rpm]
  VTQD_ActAPSPosn_pct/1 -> [VTQD_ActAPSPosn_pct]
  VTQD_RollRegenEnable_flg/1 -> [VTQD_RollRegenEnable_flg]
  VTQD_RollingShaftSpd_rpm/1 -> [VTQD_RollingShaftSpd_rpm]
  [VTQD_RollRegenEnable_flg] -> Switch/2
  [VTQD_RollGenMapEL1_Nm] -> Switch/1
  [VTQD_ECOTqMapD_Nm] -> Switch/3
  Switch/1 -> VTQD_ELTqMapDOutInv_Nm/1

== system tqdtqr_rebuild_V3/Input_Convert/Main function/DriverWhlTqDem function/Driver mode determination/NOLHM ShiftD ECO LV1  ==
  VTQD_RollRegenEnable_flg : Inport
  VTQD_RollingShaftSpd_rpm : Inport  Port=2
  VTQD_TqTargetShaftSpd_rpm : Inport  Port=3
  VTQD_ActAPSPosn_pct : Inport  Port=4
  VTQD_RL1TqMapDComp_Nm : Inport  Port=5
  Enable : EnablePort
  Add : Sum
  MTQD_ECOTqMapD_Z_Nm : Lookup_n-D  BreakpointsForDimension1=ATQD_ECOTqMapD_Y_pct  BreakpointsForDimension2=ATQD_ECOTqMapD_X_rpm  Table=MTQD_ECOTqMapD_Z_Nm  ExtrapMethod=Clip  InternalRulePriority=Speed  RndMeth=Simplest  InputSameDT=on
      settings: InputPortMap=u0,u1
  MTQD_RollGenMapEL1_Z_Nm : Lookup_n-D  BreakpointsForDimension1=ATQD_RollGenMapEL1_Y_rpm  BreakpointsForDimension2=ATQD_RollGenMapEL1_X_rpm  Table=MTQD_RollGenMapEL1_Z_Nm  ExtrapMethod=Clip  InternalRulePriority=Speed  RndMeth=Simplest  InputSameDT=on
      settings: InputPortMap=u0,u1
  Switch : Switch  Criteria=u2 ~= 0
      settings: AttributesFormatString=%<Criteria>
  VTQD_EL1TqMapDOut_Nm : Outport
  wires:
  MTQD_RollGenMapEL1_Z_Nm/1 -> [VTQD_RollGenMapEL1_Nm]
  [VTQD_RollingShaftSpd_rpm] -> MTQD_RollGenMapEL1_Z_Nm/1
  [VTQD_ActAPSPosn_pct] -> MTQD_ECOTqMapD_Z_Nm/1
  [VTQD_TqTargetShaftSpd_rpm] -> MTQD_ECOTqMapD_Z_Nm/2
  [VTQD_TqTargetShaftSpd_rpm] -> MTQD_RollGenMapEL1_Z_Nm/2
  MTQD_ECOTqMapD_Z_Nm/1 -> [VTQD_ECOTqMapD_Nm]
  VTQD_ActAPSPosn_pct/1 -> [VTQD_ActAPSPosn_pct]
  VTQD_RollingShaftSpd_rpm/1 -> [VTQD_RollingShaftSpd_rpm]
  VTQD_TqTargetShaftSpd_rpm/1 -> [VTQD_TqTargetShaftSpd_rpm]
  VTQD_RollRegenEnable_flg/1 -> [VTQD_RollRegenEnable_flg]
  [VTQD_RollRegenEnable_flg] -> Switch/2
  [VTQD_RollGenMapEL1_Nm] -> Switch/1
  [VTQD_ECOTqMapD_Nm] -> Switch/3
  Switch/1 -> Add/1
  [VTQD_RL1TqMapDComp_Nm] -> Add/2
  Add/1 -> VTQD_EL1TqMapDOut_Nm/1
  VTQD_RL1TqMapDComp_Nm/1 -> [VTQD_RL1TqMapDComp_Nm]

== system tqdtqr_rebuild_V3/Input_Convert/Main function/DriverWhlTqDem function/Driver mode determination/NOLHM ShiftD ECO LV2 ==
  VTQD_ActAPSPosn_pct : Inport
  VTQD_TqTargetShaftSpd_rpm : Inport  Port=2
  VTQD_RL2TqMapDComp_Nm : Inport  Port=3
  Enable : EnablePort
  Add : Sum
  MTQD_EL2TqMapD_Z_Nm : Lookup_n-D  BreakpointsForDimension1=ATQD_ECOTqMapD_Y_pct  BreakpointsForDimension2=ATQD_ECOTqMapD_X_rpm  Table=MTQD_EL2TqMapD_Z_Nm  ExtrapMethod=Clip  InternalRulePriority=Speed  RndMeth=Simplest  InputSameDT=on
      settings: InputPortMap=u0,u1
  VTQD_EL2TqMapDOut_Nm : Outport
  wires:
  [VTQD_TqTargetShaftSpd_rpm] -> MTQD_EL2TqMapD_Z_Nm/2
  [VTQD_ActAPSPosn_pct] -> MTQD_EL2TqMapD_Z_Nm/1
  MTQD_EL2TqMapD_Z_Nm/1 -> [VTQD_EL2TqMapD_Nm]
  VTQD_TqTargetShaftSpd_rpm/1 -> [VTQD_TqTargetShaftSpd_rpm]
  VTQD_ActAPSPosn_pct/1 -> [VTQD_ActAPSPosn_pct]
  [VTQD_EL2TqMapD_Nm] -> Add/1
  [VTQD_RL2TqMapDComp_Nm] -> Add/2
  Add/1 -> VTQD_EL2TqMapDOut_Nm/1
  VTQD_RL2TqMapDComp_Nm/1 -> [VTQD_RL2TqMapDComp_Nm]

== system tqdtqr_rebuild_V3/Input_Convert/Main function/DriverWhlTqDem function/Driver mode determination/NOLHM ShiftD ECO LV3 ==
  VTQD_ActAPSPosn_pct : Inport
  VTQD_TqTargetShaftSpd_rpm : Inport  Port=2
  VTQD_RL3TqMapDComp_Nm : Inport  Port=3
  Enable : EnablePort
  Add : Sum
  MTQD_EL3TqMapD_Z_Nm : Lookup_n-D  BreakpointsForDimension1=ATQD_ECOTqMapD_Y_pct  BreakpointsForDimension2=ATQD_ECOTqMapD_X_rpm  Table=MTQD_EL3TqMapD_Z_Nm  ExtrapMethod=Clip  InternalRulePriority=Speed  RndMeth=Simplest  InputSameDT=on
      settings: InputPortMap=u0,u1
  VTQD_EL3TqMapDOut_Nm : Outport
  wires:
  [VTQD_TqTargetShaftSpd_rpm] -> MTQD_EL3TqMapD_Z_Nm/2
  [VTQD_ActAPSPosn_pct] -> MTQD_EL3TqMapD_Z_Nm/1
  MTQD_EL3TqMapD_Z_Nm/1 -> [VTQD_EL3TqMapD_Nm]
  VTQD_TqTargetShaftSpd_rpm/1 -> [VTQD_TqTargetShaftSpd_rpm]
  VTQD_ActAPSPosn_pct/1 -> [VTQD_ActAPSPosn_pct]
  [VTQD_RL3TqMapDComp_Nm] -> Add/1
  [VTQD_EL3TqMapD_Nm] -> Add/2
  Add/1 -> VTQD_EL3TqMapDOut_Nm/1
  VTQD_RL3TqMapDComp_Nm/1 -> [VTQD_RL3TqMapDComp_Nm]

== system tqdtqr_rebuild_V3/Input_Convert/Main function/DriverWhlTqDem function/Driver mode determination/NOLHM ShiftD ECO LV4 ==
  VTQD_ActAPSPosn_pct : Inport
  VTQD_TqTargetShaftSpd_rpm : Inport  Port=2
  VTQD_RL4TqMapDComp_Nm : Inport  Port=3
  Enable : EnablePort
  Add : Sum
  MTQD_EL4TqMapD_Z_Nm : Lookup_n-D  BreakpointsForDimension1=ATQD_ECOTqMapD_Y_pct  BreakpointsForDimension2=ATQD_ECOTqMapD_X_rpm  Table=MTQD_EL4TqMapD_Z_Nm  ExtrapMethod=Clip  InternalRulePriority=Speed  RndMeth=Simplest  InputSameDT=on
      settings: InputPortMap=u0,u1
  VTQD_EL4TqMapDOut_Nm : Outport
  wires:
  MTQD_EL4TqMapD_Z_Nm/1 -> [VTQD_EL4TqMapD_Nm]
  [VTQD_ActAPSPosn_pct] -> MTQD_EL4TqMapD_Z_Nm/1
  [VTQD_TqTargetShaftSpd_rpm] -> MTQD_EL4TqMapD_Z_Nm/2
  VTQD_TqTargetShaftSpd_rpm/1 -> [VTQD_TqTargetShaftSpd_rpm]
  VTQD_ActAPSPosn_pct/1 -> [VTQD_ActAPSPosn_pct]
  [VTQD_RL4TqMapDComp_Nm] -> Add/1
  [VTQD_EL4TqMapD_Nm] -> Add/2
  Add/1 -> VTQD_EL4TqMapDOut_Nm/1
  VTQD_RL4TqMapDComp_Nm/1 -> [VTQD_RL4TqMapDComp_Nm]

== system tqdtqr_rebuild_V3/Input_Convert/Main function/DriverWhlTqDem function/Driver mode determination/NOLHM ShiftD ECO LV5 ==
  VTQD_ActAPSPosn_pct : Inport
  VTQD_TqTargetShaftSpd_rpm : Inport  Port=2
  VTQD_RL5TqMapDComp_Nm : Inport  Port=3
  Enable : EnablePort
  Add : Sum
  MTQD_EL5TqMapD_Z_Nm : Lookup_n-D  BreakpointsForDimension1=ATQD_ECOTqMapD_Y_pct  BreakpointsForDimension2=ATQD_ECOTqMapD_X_rpm  Table=MTQD_EL5TqMapD_Z_Nm  ExtrapMethod=Clip  InternalRulePriority=Speed  RndMeth=Simplest  InputSameDT=on
      settings: InputPortMap=u0,u1
  VTQD_EL5TqMapDOut_Nm : Outport
  wires:
  [VTQD_TqTargetShaftSpd_rpm] -> MTQD_EL5TqMapD_Z_Nm/2
  [VTQD_ActAPSPosn_pct] -> MTQD_EL5TqMapD_Z_Nm/1
  MTQD_EL5TqMapD_Z_Nm/1 -> [VTQD_EL5TqMapD_Nm]
  VTQD_ActAPSPosn_pct/1 -> [VTQD_ActAPSPosn_pct]
  VTQD_TqTargetShaftSpd_rpm/1 -> [VTQD_TqTargetShaftSpd_rpm]
  [VTQD_RL5TqMapDComp_Nm] -> Add/1
  [VTQD_EL5TqMapD_Nm] -> Add/2
  Add/1 -> VTQD_EL5TqMapDOut_Nm/1
  VTQD_RL5TqMapDComp_Nm/1 -> [VTQD_RL5TqMapDComp_Nm]

== system tqdtqr_rebuild_V3/Input_Convert/Main function/DriverWhlTqDem function/Driver mode determination/NOLHM ShiftD ECO OPD ==
  VTQD_ActAPSPosn_pct : Inport
  VTQD_TqTargetShaftSpd_rpm : Inport  Port=2
  VVMC_EstSlope_Deg : Inport  Port=3
  VTQD_APSReqTimer_s : Inport  Port=4
  VTQD_LowIdleAccPedal_flg : Inport  Port=5
  VTQD_OPDHoldEnRel_flg : Inport  Port=6
  VTQD_OPDHoldActRelTq_Nm : Inport  Port=7
  VTQD_VehActSpd_kph : Inport  Port=8
  VTQD_SlopeUp_flg : Inport  Port=9
  Enable : EnablePort
  AND : Logic  AllPortsSameDT=off  OutDataTypeStr=boolean
  Add : Sum
  Constant1 : Constant  Value=ZERO_FLOAT
  Constant2 : Constant  Value=KTQD_OPDHTqDisComSpd_kph
  Constant3 : Constant  Value=KTQD_OPDHTqDisAPSPosn_pct
  Constant9 : Constant  Value=KTQD_APSReqDelayTime_s
  Detect Increase : simulink/Logic and Bit Operations/Detect Increase  vinit=0.0  OutDataTypeStr=boolean
  MTQD_EOPDTqMapDCon_Z_Nm : Lookup_n-D  BreakpointsForDimension1=ATQD_EOPDTqMapDCon_Y_Deg  BreakpointsForDimension2=ATQD_EOPDTqMapDCon_X_rpm  Table=MTQD_EOPDTqMapDCon_Z_Nm  ExtrapMethod=Clip  InternalRulePriority=Speed  RndMeth=Simplest  InputSameDT=on
      settings: InputPortMap=u0,u1
  MTQD_EOPDTqMapD_Z_Nm : Lookup_n-D  BreakpointsForDimension1=ATQD_ECOTqMapD_Y_pct  BreakpointsForDimension2=ATQD_ECOTqMapD_X_rpm  Table=MTQD_EOPDTqMapD_Z_Nm  ExtrapMethod=Clip  InternalRulePriority=Speed  RndMeth=Simplest  InputSameDT=on
      settings: InputPortMap=u0,u1
  Max : MinMax  Function=max  Inputs=2
  NOT : Logic  Operator=NOT  AllPortsSameDT=off  OutDataTypeStr=boolean
  OR : Logic  Operator=OR  Inputs=3  AllPortsSameDT=off  OutDataTypeStr=boolean
  OR1 : Logic  Operator=OR  AllPortsSameDT=off  OutDataTypeStr=boolean
  Relational Operator : RelationalOperator  Operator=>  OutDataTypeStr=boolean  RndMeth=Simplest
  Relational Operator1 : RelationalOperator  OutDataTypeStr=boolean  RndMeth=Simplest
  Relational Operator2 : RelationalOperator  OutDataTypeStr=boolean  RndMeth=Simplest
  SR_Latch : hcu_lib/Basic_Blocks/SR_Latch
  Switch : Switch  Criteria=u2 ~= 0
      settings: AttributesFormatString=%<Criteria>
  Switch1 : Switch  Criteria=u2 ~= 0
      settings: AttributesFormatString=%<Criteria>
  VTQD_EOPDTqMapDOut_Nm : Outport
  wires:
  MTQD_EOPDTqMapD_Z_Nm/1 -> [VTQD_EOPDTqMapD_Nm]
  [VTQD_TqTargetShaftSpd_rpm] -> MTQD_EOPDTqMapD_Z_Nm/2
  [VVMC_EstSlope_Deg] -> MTQD_EOPDTqMapDCon_Z_Nm/1
  MTQD_EOPDTqMapDCon_Z_Nm/1 -> [VTQD_EOPDTqMapDCon_Nm]
  [VTQD_ActAPSPosn_pct] -> MTQD_EOPDTqMapD_Z_Nm/1
  [VTQD_TqTargetShaftSpd_rpm] -> MTQD_EOPDTqMapDCon_Z_Nm/2
  VVMC_EstSlope_Deg/1 -> [VVMC_EstSlope_Deg]
  VTQD_ActAPSPosn_pct/1 -> [VTQD_ActAPSPosn_pct]
  VTQD_TqTargetShaftSpd_rpm/1 -> [VTQD_TqTargetShaftSpd_rpm]
  [VTQD_APSReqTimer_s] -> Relational Operator2/1
  Constant3/1 -> Relational Operator1/2
  [VTQD_LowIdleAccPedal_flg] -> AND/2
  Constant1/1 -> Switch/1
  AND/1 -> OR1/1
  OR1/1 -> Switch/2
  Constant9/1 -> Relational Operator2/2
  Switch/1 -> Add/2
  Relational Operator2/1 -> AND/1
  [VTQD_ActAPSPosn_pct] -> Relational Operator1/1
  Relational Operator1/1 -> OR1/2
  [VTQD_EOPDTqMapD_Nm] -> Add/1
  [VTQD_EOPDTqMapDCon_Nm] -> Switch/3
  VTQD_APSReqTimer_s/1 -> [VTQD_APSReqTimer_s]
  VTQD_LowIdleAccPedal_flg/1 -> [VTQD_LowIdleAccPedal_flg]
  VTQD_OPDHoldEnRel_flg/1 -> [VTQD_OPDHoldEnRel_flg]
  VTQD_OPDHoldActRelTq_Nm/1 -> [VTQD_OPDHoldActRelTq_Nm]
  VTQD_VehActSpd_kph/1 -> [VTQD_VehActSpd_kph]
  VTQD_SlopeUp_flg/1 -> [VTQD_SlopeUp_flg]
  SR_Latch/1 -> Switch1/2
  Relational Operator/1 -> OR/2
  OR/1 -> SR_Latch/2
  Add/1 -> Switch1/3, Max/1  "VTQD_EOPDActTqMapD_Nm"
  Max/1 -> Switch1/1
  [VTQD_OPDHoldEnRel_flg] -> Detect Increase/1
  [VTQD_OPDHoldActRelTq_Nm] -> Max/2
  NOT/1 -> OR/3
  Constant2/1 -> Relational Operator/2
  Switch1/1 -> VTQD_EOPDTqMapDOut_Nm/1
  [VTQD_LowIdleAccPedal_flg] -> OR/1
  Detect Increase/1 -> SR_Latch/1
  [VTQD_VehActSpd_kph] -> Relational Operator/1
  [VTQD_SlopeUp_flg] -> NOT/1

== system tqdtqr_rebuild_V3/Input_Convert/Main function/DriverWhlTqDem function/Driver mode determination/NOLHM ShiftD NRM Invalid ==
  VTQD_ActAPSPosn_pct : Inport
  VTQD_TqTargetShaftSpd_rpm : Inport  Port=2
  Enable : EnablePort
  MTQD_NL1TqMapD_Z_Nm : Lookup_n-D  BreakpointsForDimension1=ATQD_NL1TqMapD_Y_pct  BreakpointsForDimension2=ATQD_NL1TqMapD_X_rpm  Table=MTQD_NL1TqMapD_Z_Nm  ExtrapMethod=Clip  InternalRulePriority=Speed  RndMeth=Simplest  InputSameDT=on
      settings: InputPortMap=u0,u1
  VTQD_NLTqMapDOutInv_Nm : Outport
  wires:
  MTQD_NL1TqMapD_Z_Nm/1 -> [VTQD_NL1TqMapD_Nm]
  [VTQD_TqTargetShaftSpd_rpm] -> MTQD_NL1TqMapD_Z_Nm/2
  [VTQD_ActAPSPosn_pct] -> MTQD_NL1TqMapD_Z_Nm/1
  VTQD_ActAPSPosn_pct/1 -> [VTQD_ActAPSPosn_pct]
  VTQD_TqTargetShaftSpd_rpm/1 -> [VTQD_TqTargetShaftSpd_rpm]
  [VTQD_NL1TqMapD_Nm] -> VTQD_NLTqMapDOutInv_Nm/1

== system tqdtqr_rebuild_V3/Input_Convert/Main function/DriverWhlTqDem function/Driver mode determination/NOLHM ShiftD NRM LV1 ==
  VTQD_ActAPSPosn_pct : Inport
  VTQD_TqTargetShaftSpd_rpm : Inport  Port=2
  VTQD_RL1TqMapDComp_Nm : Inport  Port=3
  Enable : EnablePort
  Add : Sum
  MTQD_NL1TqMapD_Z_Nm : Lookup_n-D  BreakpointsForDimension1=ATQD_NL1TqMapD_Y_pct  BreakpointsForDimension2=ATQD_NL1TqMapD_X_rpm  Table=MTQD_NL1TqMapD_Z_Nm  ExtrapMethod=Clip  InternalRulePriority=Speed  RndMeth=Simplest  InputSameDT=on
      settings: InputPortMap=u0,u1
  VTQD_NL1TqMapDOut_Nm : Outport
  wires:
  MTQD_NL1TqMapD_Z_Nm/1 -> [VTQD_NL1TqMapD_Nm]
  [VTQD_TqTargetShaftSpd_rpm] -> MTQD_NL1TqMapD_Z_Nm/2
  [VTQD_ActAPSPosn_pct] -> MTQD_NL1TqMapD_Z_Nm/1
  VTQD_ActAPSPosn_pct/1 -> [VTQD_ActAPSPosn_pct]
  VTQD_TqTargetShaftSpd_rpm/1 -> [VTQD_TqTargetShaftSpd_rpm]
  [VTQD_NL1TqMapD_Nm] -> Add/2
  [VTQD_RL1TqMapDComp_Nm] -> Add/1
  Add/1 -> VTQD_NL1TqMapDOut_Nm/1
  VTQD_RL1TqMapDComp_Nm/1 -> [VTQD_RL1TqMapDComp_Nm]

== system tqdtqr_rebuild_V3/Input_Convert/Main function/DriverWhlTqDem function/Driver mode determination/NOLHM ShiftD NRM LV2 ==
  VTQD_ActAPSPosn_pct : Inport
  VTQD_TqTargetShaftSpd_rpm : Inport  Port=2
  VTQD_RL2TqMapDComp_Nm : Inport  Port=3
  Enable : EnablePort
  Add : Sum
  MTQD_NL2TqMapD_Z_Nm : Lookup_n-D  BreakpointsForDimension1=ATQD_NL1TqMapD_Y_pct  BreakpointsForDimension2=ATQD_NL1TqMapD_X_rpm  Table=MTQD_NL2TqMapD_Z_Nm  ExtrapMethod=Clip  InternalRulePriority=Speed  RndMeth=Simplest  InputSameDT=on
      settings: InputPortMap=u0,u1
  VTQD_NL2TqMapDOut_Nm : Outport
  wires:
  [VTQD_TqTargetShaftSpd_rpm] -> MTQD_NL2TqMapD_Z_Nm/2
  MTQD_NL2TqMapD_Z_Nm/1 -> [VTQD_NL2TqMapD_Nm]
  [VTQD_ActAPSPosn_pct] -> MTQD_NL2TqMapD_Z_Nm/1
  VTQD_ActAPSPosn_pct/1 -> [VTQD_ActAPSPosn_pct]
  VTQD_TqTargetShaftSpd_rpm/1 -> [VTQD_TqTargetShaftSpd_rpm]
  [VTQD_RL2TqMapDComp_Nm] -> Add/1
  [VTQD_NL2TqMapD_Nm] -> Add/2
  Add/1 -> VTQD_NL2TqMapDOut_Nm/1
  VTQD_RL2TqMapDComp_Nm/1 -> [VTQD_RL2TqMapDComp_Nm]

== system tqdtqr_rebuild_V3/Input_Convert/Main function/DriverWhlTqDem function/Driver mode determination/NOLHM ShiftD NRM LV3 ==
  VTQD_ActAPSPosn_pct : Inport
  VTQD_TqTargetShaftSpd_rpm : Inport  Port=2
  VTQD_RL3TqMapDComp_Nm : Inport  Port=3
  Enable : EnablePort
  Add : Sum
  MTQD_NL3TqMapD_Z_Nm : Lookup_n-D  BreakpointsForDimension1=ATQD_NL1TqMapD_Y_pct  BreakpointsForDimension2=ATQD_NL1TqMapD_X_rpm  Table=MTQD_NL3TqMapD_Z_Nm  ExtrapMethod=Clip  InternalRulePriority=Speed  RndMeth=Simplest  InputSameDT=on
      settings: InputPortMap=u0,u1
  VTQD_NL3TqMapDOut_Nm : Outport
  wires:
  VTQD_TqTargetShaftSpd_rpm/1 -> [VTQD_TqTargetShaftSpd_rpm]
  [VTQD_ActAPSPosn_pct] -> MTQD_NL3TqMapD_Z_Nm/1
  [VTQD_TqTargetShaftSpd_rpm] -> MTQD_NL3TqMapD_Z_Nm/2
  MTQD_NL3TqMapD_Z_Nm/1 -> [VTQD_NL3TqMapD_Nm]
  VTQD_ActAPSPosn_pct/1 -> [VTQD_ActAPSPosn_pct]
  [VTQD_RL3TqMapDComp_Nm] -> Add/1
  [VTQD_NL3TqMapD_Nm] -> Add/2
  Add/1 -> VTQD_NL3TqMapDOut_Nm/1
  VTQD_RL3TqMapDComp_Nm/1 -> [VTQD_RL3TqMapDComp_Nm]

== system tqdtqr_rebuild_V3/Input_Convert/Main function/DriverWhlTqDem function/Driver mode determination/NOLHM ShiftD NRM LV4 ==
  VTQD_ActAPSPosn_pct : Inport
  VTQD_TqTargetShaftSpd_rpm : Inport  Port=2
  VTQD_RL4TqMapDComp_Nm : Inport  Port=3
  Enable : EnablePort
  Add : Sum
  MTQD_NL4TqMapD_Z_Nm1 : Lookup_n-D  BreakpointsForDimension1=ATQD_NL1TqMapD_Y_pct  BreakpointsForDimension2=ATQD_NL1TqMapD_X_rpm  Table=MTQD_NL4TqMapD_Z_Nm  ExtrapMethod=Clip  InternalRulePriority=Speed  RndMeth=Simplest  InputSameDT=on
      settings: InputPortMap=u0,u1
  VTQD_NL4TqMapDOut_Nm : Outport
  wires:
  [VTQD_TqTargetShaftSpd_rpm] -> MTQD_NL4TqMapD_Z_Nm1/2
  MTQD_NL4TqMapD_Z_Nm1/1 -> [VTQD_NL4TqMapD_Nm]
  [VTQD_ActAPSPosn_pct] -> MTQD_NL4TqMapD_Z_Nm1/1
  VTQD_ActAPSPosn_pct/1 -> [VTQD_ActAPSPosn_pct]
  VTQD_TqTargetShaftSpd_rpm/1 -> [VTQD_TqTargetShaftSpd_rpm]
  [VTQD_NL4TqMapD_Nm] -> Add/1
  [VTQD_RL4TqMapDComp_Nm] -> Add/2
  Add/1 -> VTQD_NL4TqMapDOut_Nm/1
  VTQD_RL4TqMapDComp_Nm/1 -> [VTQD_RL4TqMapDComp_Nm]
